simulink model "p3_model"  (Simulink 8.7)
settings: Solver=FixedStepAuto  StartTime=0.0  StopTime=1.0  FixedStep=0.001  RelTol=1e-3
libraries: simulink x1
settings Model: Creator=eispin  LastModifiedBy=eispin
settings DataIOCC: LimitDataPoints=off  SaveFormat=Dataset
settings DebuggingCC: UnderspecifiedInitializationDetection=Simplified  MergeDetectMultiDrivingBlocksExec=error
settings HardwareCC: ProdBitPerPointer=64  ProdLargestAtomicFloat=Float  ProdIntDivRoundTo=Zero  ProdEndianess=LittleEndian  ProdWordSize=64  ProdHWDeviceType=Intel->x86-64 (Windows64)
settings ModelReferenceCC: PropagateSignalLabelsOutOfModel=on
settings ConfigComp: CovModelRefEnable=off

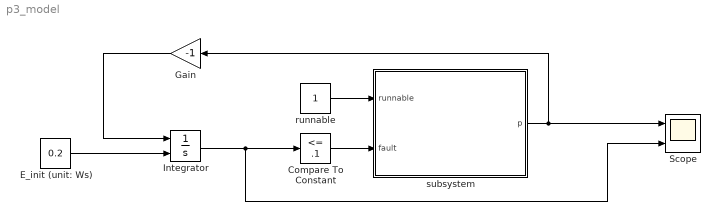
== system p3_model ==
  Compare To Constant : simulink/Logic and Bit Operations/Compare To Constant  relop=<=  const=.1  OutDataTypeStr=boolean
  E_init (unit: Ws) : Constant  Value=0.2
  Gain : Gain  Gain=-1
  Integrator : Integrator  InitialConditionSource=external
  Scope : Scope  NumInputPorts=2
  runnable : Constant
  subsystem : Stateflow chart  TreatAsAtomicUnit=on
  wires:
  E_init (unit: Ws)/1 -> Integrator/2
  runnable/1 -> subsystem/1(runnable)
  Compare To Constant/1 -> subsystem/2(fault)
  subsystem/1(p) -> Scope/1, Gain/1
  Integrator/1 -> Scope/2, Compare To Constant/1
  Gain/1 -> Integrator/1

== stateflow chart subsystem ==
  state RUN
    entry:
    p=.4
  state IDLE
    entry:
    p=.05
  state SLEEP
    entry:
    p=.000160
  (default) -> RUN
  RUN -> IDLE [order 1] : [fault < .5 && after(10,usec)]
  RUN -> SLEEP [order 2] : [fault > .5 && after(90,usec)]
  IDLE -> RUN [order 1] : [fault < .5 && runnable > .5 && after(10, usec)]
  SLEEP -> RUN : [runnable > .5 && after(160,msec)]
  IDLE -> SLEEP [order 2] : [fault > .5 && after(90, usec)]
  data: runnable input double; fault input double; p output double
